simulink model "Critically_Damped_SMD_System__1_"  (R2023b)
settings: Solver=VariableStepAuto  StartTime=0.0  StopTime=10  RelTol=1e-3
settings Model: Creator=91839  LastModifiedBy=siva kumar
settings SolverCC: AlgebraicLoopSolver=TrustRegion
settings DataIOCC: ExternalInput=data  SaveFormat=Array  DSMLogging=off  ReturnWorkspaceOutputs=off
settings DebuggingCC: UnconnectedInputMsg=warning  UnconnectedOutputMsg=warning  UnconnectedLineMsg=warning
settings ModelReferenceCC: EnableRefExpFcnMdlSchedulingChecks=on
settings SFSimCC: CustomCodeUndefinedFunction=UseInterfaceOnly

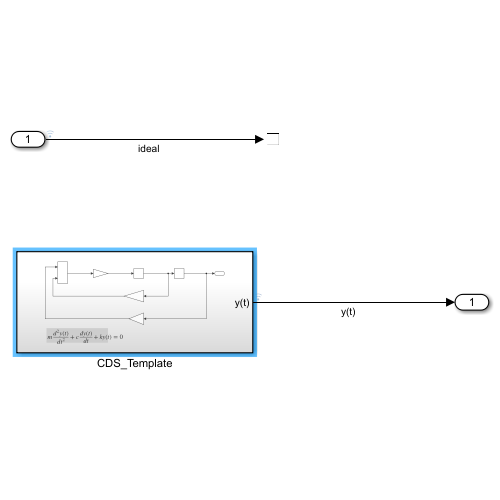
[thumbnail: Simulink's stored preview of the top-level diagram]
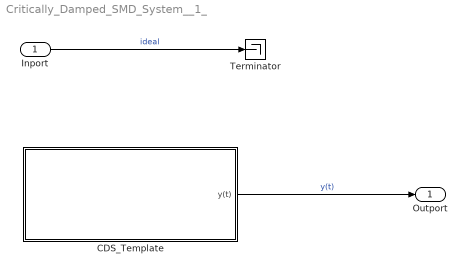
== system Critically_Damped_SMD_System__1_ ==
  Inport : Inport
  CDS_Template : Subsystem
  Terminator : Terminator
  Outport : Outport
  wires:
  Inport/1 -> Terminator/1  "ideal"
  CDS_Template/1(y(t)) -> Outport/1  "y(t)"

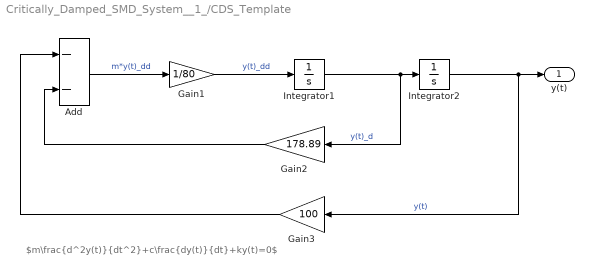
== system Critically_Damped_SMD_System__1_/CDS_Template ==
  note: $m\frac{d^2y(t)}{dt^2}+c\frac{dy(t)}{dt}+ky(t)=0$
  Add : Sum  Inputs=--
  Gain1 : Gain  Gain=1/80
  Gain2 : Gain  Gain=178.89
  Gain3 : Gain  Gain=100
  Integrator1 : Integrator
  Integrator2 : Integrator  InitialCondition=2
  y(t) : Outport
  wires:
  Add/1 -> Gain1/1  "m*y(t)_dd"
  Gain1/1 -> Integrator1/1  "y(t)_dd"
  Integrator1/1 -> Gain2/1, Integrator2/1  "y(t)_d"
  Integrator2/1 -> Gain3/1, y(t)/1  "y(t)"
  Gain2/1 -> Add/2
  Gain3/1 -> Add/1
